simulink model "PID_miniHopper_5_Pitch_Roll_Yaw_Contour_5_full"  (R2022b)
settings: Solver=VariableStepAuto  StartTime=0.0  StopTime=10  RelTol=1e-3
values from neighbouring files (symbols this model uses):
  hopper_ode = struct()    [MiniHopperParameters.m]
undefined symbols (not defined in the file or in its folder): A_alt, A_rpy, B_alt, B_rpy, Gain_pitch_U, Gain_roll_U, Gain_yaw_U, kT, VxLoop, VyLoop, XIC_rpy, XLoop, YLoop
libraries: simulink_extras x16, slpidlib x12
(part 2 of 2)

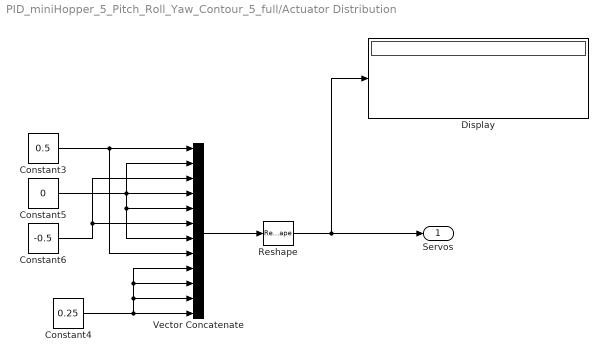
== system PID_miniHopper_5_Pitch_Roll_Yaw_Contour_5_full/Actuator Distribution ==
  Constant3 : Constant  Value=0.5
  Constant4 : Constant  Value=0.25
  Constant5 : Constant  Value=0
  Constant6 : Constant  Value=-0.5
  Display : Display
  Reshape : Reshape  OutputDimensionality=Customize  OutputDimensions=[4,3]
  Vector Concatenate : Concatenate  NumInputs=12
  Servos : Outport
  wires:
  Constant5/1 -> Vector Concatenate/7, Vector Concatenate/5, Vector Concatenate/4, Vector Concatenate/2
  Constant6/1 -> Vector Concatenate/6, Vector Concatenate/3
  Constant3/1 -> Vector Concatenate/8, Vector Concatenate/1
  Constant4/1 -> Vector Concatenate/9, Vector Concatenate/10, Vector Concatenate/11, Vector Concatenate/12
  Reshape/1 -> Servos/1, Display/1
  Vector Concatenate/1 -> Reshape/1

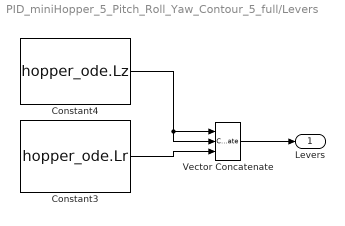
== system PID_miniHopper_5_Pitch_Roll_Yaw_Contour_5_full/Levers ==
  Constant3 : Constant  Value=hopper_ode.Lr
  Constant4 : Constant  Value=hopper_ode.Lz
  Vector Concatenate : Concatenate  NumInputs=3
  Levers : Outport
  wires:
  Constant4/1 -> Vector Concatenate/2, Vector Concatenate/1
  Constant3/1 -> Vector Concatenate/3
  Vector Concatenate/1 -> Levers/1

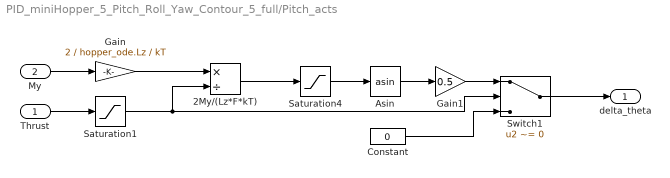
== system PID_miniHopper_5_Pitch_Roll_Yaw_Contour_5_full/Pitch_acts ==
  Thrust : Inport
  My : Inport  Port=2
  2My/(Lz*F*kT) : Product  Inputs=*/
  Asin : Trigonometry  Operator=asin
  Constant : Constant  Value=0
  Gain : Gain  Gain=2 / hopper_ode.Lz / kT
  Gain1 : Gain  Gain=0.5
  Saturation1 : Saturate  UpperLimit=25  LowerLimit=0
  Saturation4 : Saturate  UpperLimit=1  LowerLimit=-1
  Switch1 : Switch  Criteria=u2 ~= 0  SaturateOnIntegerOverflow=off  InputSameDT=off
  delta_theta : Outport
  wires:
  Gain/1 -> 2My/(Lz*F*kT)/1
  Switch1/1 -> delta_theta/1
  Constant/1 -> Switch1/3
  Thrust/1 -> Saturation1/1
  Saturation1/1 -> Switch1/2, 2My/(Lz*F*kT)/2
  Asin/1 -> Gain1/1
  Saturation4/1 -> Asin/1
  My/1 -> Gain/1
  2My/(Lz*F*kT)/1 -> Saturation4/1
  Gain1/1 -> Switch1/1

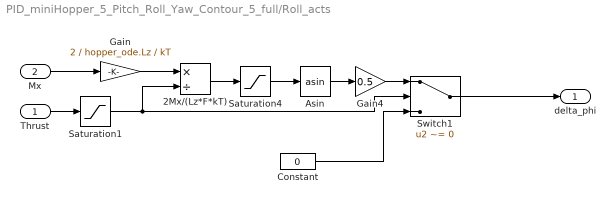
== system PID_miniHopper_5_Pitch_Roll_Yaw_Contour_5_full/Roll_acts ==
  Thrust : Inport
  Mx : Inport  Port=2
  2Mx/(Lz*F*kT) : Product  Inputs=*/
  Asin : Trigonometry  Operator=asin
  Constant : Constant  Value=0
  Gain : Gain  Gain=2 / hopper_ode.Lz / kT
  Gain4 : Gain  Gain=0.5
  Saturation1 : Saturate  UpperLimit=25  LowerLimit=0
  Saturation4 : Saturate  UpperLimit=1  LowerLimit=-1
  Switch1 : Switch  Criteria=u2 ~= 0  SaturateOnIntegerOverflow=off  InputSameDT=off
  delta_phi : Outport
  wires:
  Saturation4/1 -> Asin/1
  Asin/1 -> Gain4/1
  Saturation1/1 -> Switch1/2, 2Mx/(Lz*F*kT)/2
  Thrust/1 -> Saturation1/1
  Constant/1 -> Switch1/3
  Switch1/1 -> delta_phi/1
  2Mx/(Lz*F*kT)/1 -> Saturation4/1
  Gain/1 -> 2Mx/(Lz*F*kT)/1
  Mx/1 -> Gain/1
  Gain4/1 -> Switch1/1

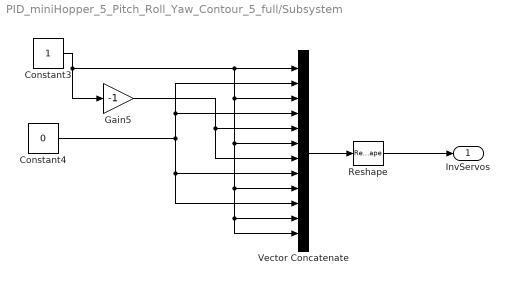
== system PID_miniHopper_5_Pitch_Roll_Yaw_Contour_5_full/Subsystem ==
  Constant3 : Constant
  Constant4 : Constant  Value=0
  Gain5 : Gain  Gain=-1
  Reshape : Reshape  OutputDimensionality=Customize  OutputDimensions=[3,4]
  Vector Concatenate : Concatenate  NumInputs=12
  InvServos : Outport
  wires:
  Constant3/1 -> Vector Concatenate/1, Vector Concatenate/12, Vector Concatenate/11, Vector Concatenate/9, Vector Concatenate/6, Vector Concatenate/3, Gain5/1
  Constant4/1 -> Vector Concatenate/2, Vector Concatenate/4, Vector Concatenate/10, Vector Concatenate/8
  Vector Concatenate/1 -> Reshape/1
  Gain5/1 -> Vector Concatenate/7, Vector Concatenate/5
  Reshape/1 -> InvServos/1

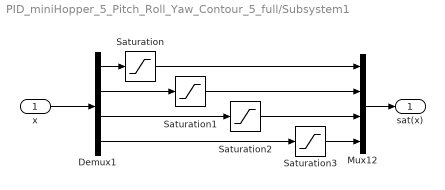
== system PID_miniHopper_5_Pitch_Roll_Yaw_Contour_5_full/Subsystem1 ==
  x : Inport
  Demux1 : Demux
  Mux12 : Mux
  Saturation{,1..3} (4 alike) : Saturate  UpperLimit=deg2rad(45)  LowerLimit=-deg2rad(45)
  sat(x) : Outport
  wires:
  Demux1/3 -> Saturation2/1
  Demux1/4 -> Saturation3/1
  Demux1/1 -> Saturation/1
  Demux1/2 -> Saturation1/1
  x/1 -> Demux1/1
  Mux12/1 -> sat(x)/1
  Saturation/1 -> Mux12/1
  Saturation1/1 -> Mux12/2
  Saturation2/1 -> Mux12/3
  Saturation3/1 -> Mux12/4

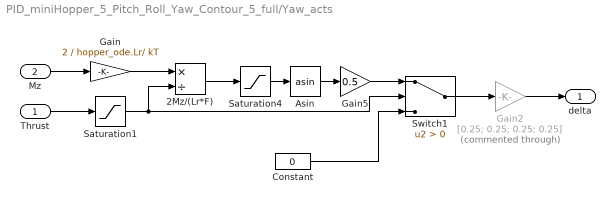
== system PID_miniHopper_5_Pitch_Roll_Yaw_Contour_5_full/Yaw_acts ==
  Thrust : Inport
  Mz : Inport  Port=2
  2Mz/(Lr*F) : Product  Inputs=*/
  Asin : Trigonometry  Operator=asin
  Constant : Constant  Value=0
  Gain : Gain  Gain=2 / hopper_ode.Lr/ kT
  Gain2 : Gain  Commented=through  Gain=[0.25; 0.25; 0.25; 0.25]
  Gain5 : Gain  Gain=0.5
  Saturation1 : Saturate  UpperLimit=25  LowerLimit=0
  Saturation4 : Saturate  UpperLimit=1  LowerLimit=-1
  Switch1 : Switch  Criteria=u2 > Threshold  SaturateOnIntegerOverflow=off  InputSameDT=off
  delta : Outport
  wires:
  Mz/1 -> Gain/1
  Gain/1 -> 2Mz/(Lr*F)/1
  2Mz/(Lr*F)/1 -> Saturation4/1
  Switch1/1 -> Gain2/1
  Constant/1 -> Switch1/3
  Thrust/1 -> Saturation1/1
  Gain2/1 -> delta/1
  Saturation1/1 -> Switch1/2, 2Mz/(Lr*F)/2
  Asin/1 -> Gain5/1
  Saturation4/1 -> Asin/1
  Gain5/1 -> Switch1/1

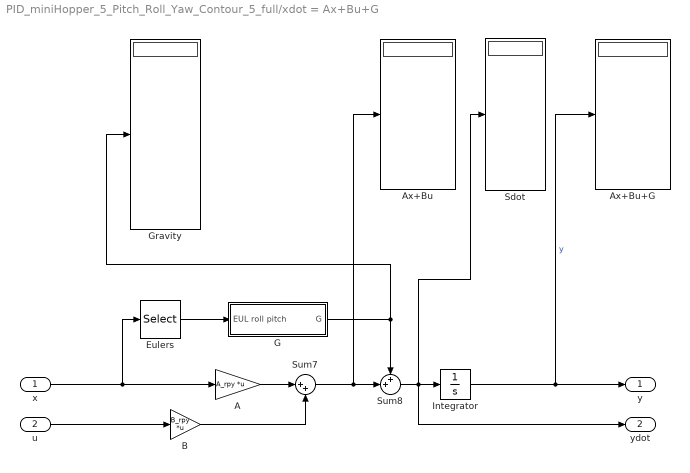
== system PID_miniHopper_5_Pitch_Roll_Yaw_Contour_5_full/xdot = Ax+Bu+G ==
  x : Inport
  u : Inport  Port=2
  A : Gain  Gain=A_rpy  Multiplication=Matrix(K*u)
  Ax+Bu : Display
  Ax+Bu+G : Display
  B : Gain  Gain=B_rpy  Multiplication=Matrix(K*u)
  Eulers : Selector  InputPortWidth=10  IndexOptions=Index vector (dialog)  Indices=[5 6 7]  OutputSizes=1
  G : Subsystem
  Gravity : Display
  Integrator : Integrator  InitialCondition=XIC_rpy
  Sdot : Display
  Sum7 : Sum  Inputs=|++
  Sum8 : Sum  Inputs=++|
  y : Outport
  ydot : Outport  Port=2
  wires:
  u/1 -> B/1
  B/1 -> Sum7/2
  Sum7/1 -> Ax+Bu/1, Sum8/2
  A/1 -> Sum7/1
  G/1(G) -> Gravity/1, Sum8/1
  x/1 -> Eulers/1, A/1
  Integrator/1 -> Ax+Bu+G/1, y/1  "y"
  Eulers/1 -> G/1(EUL roll pitch)
  Sum8/1 -> Sdot/1, ydot/1, Integrator/1

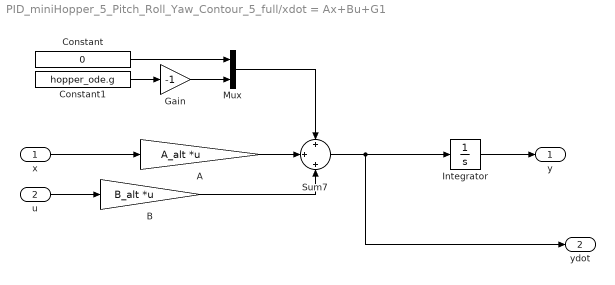
== system PID_miniHopper_5_Pitch_Roll_Yaw_Contour_5_full/xdot = Ax+Bu+G1 ==
  x : Inport
  u : Inport  Port=2
  A : Gain  Gain=A_alt  Multiplication=Matrix(K*u)
  B : Gain  Gain=B_alt  Multiplication=Matrix(K*u)
  Constant : Constant  Value=0
  Constant1 : Constant  Value=hopper_ode.g
  Gain : Gain  Gain=-1
  Integrator : Integrator  InitialCondition=[0; 0]
  Mux : Mux  Inputs=2
  Sum7 : Sum  Inputs=+|+|+
  y : Outport
  ydot : Outport  Port=2
  wires:
  u/1 -> B/1
  B/1 -> Sum7/3
  Sum7/1 -> ydot/1, Integrator/1
  A/1 -> Sum7/2
  x/1 -> A/1
  Integrator/1 -> y/1
  Constant/1 -> Mux/1
  Constant1/1 -> Gain/1
  Gain/1 -> Mux/2
  Mux/1 -> Sum7/1

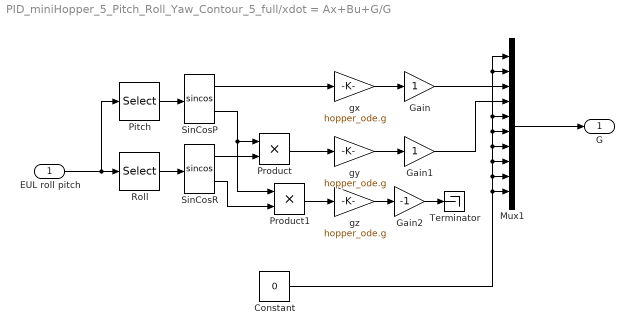
== system PID_miniHopper_5_Pitch_Roll_Yaw_Contour_5_full/xdot = Ax+Bu+G/G ==
  EUL roll pitch : Inport
  Constant : Constant  Value=0
  Gain : Gain
  Gain1 : Gain
  Gain2 : Gain  Gain=-1
  Mux1 : Mux  Inputs=10
  Pitch : Selector  InputPortWidth=3  IndexOptions=Index vector (dialog)  Indices=[2]  OutputSizes=1
  Product : Product
  Product1 : Product
  Roll : Selector  InputPortWidth=3  IndexOptions=Index vector (dialog)  Indices=[1]  OutputSizes=1
  SinCosP : Trigonometry  Operator=sincos
  SinCosR : Trigonometry  Operator=sincos
  Terminator : Terminator
  gx : Gain  Gain=hopper_ode.g
  gy : Gain  Gain=hopper_ode.g
  gz : Gain  Gain=hopper_ode.g
  G : Outport
  wires:
  Gain/1 -> Mux1/3
  Mux1/1 -> G/1
  Roll/1 -> SinCosR/1
  EUL roll pitch/1 -> Pitch/1, Roll/1
  SinCosP/2 -> Product1/1, Product/1
  SinCosR/1 -> Product/2
  gx/1 -> Gain/1
  Pitch/1 -> SinCosP/1
  SinCosP/1 -> gx/1
  Product/1 -> gy/1
  gy/1 -> Gain1/1
  Gain1/1 -> Mux1/4
  SinCosR/2 -> Product1/2
  Product1/1 -> gz/1
  gz/1 -> Gain2/1
  Gain2/1 -> Terminator/1
  Constant/1 -> Mux1/2, Mux1/1, Mux1/5, Mux1/6, Mux1/7, Mux1/8, Mux1/9, Mux1/10
